simulink model "MPC_lateralStability_IntegratedControl_DesignProgram"  (R2019b)
settings: Solver=VariableStepAuto  StartTime=0.0  StopTime=10.0  RelTol=1e-3
values from neighbouring files (symbols this model uses):
  A = [-4.40211640212  -0.830687830688; 20.8695652174  -5.1867826087]    [general_mpc_test_data.mat]
  B = [1.60846560847  0; 15.8608695652  0.000347826086957]    [general_mpc_test_data.mat]
libraries: mpclib x2
settings Model: Creator=Shouvik Chakraborty  LastModifiedBy=shouv
settings SFSimCC: CustomCodeUndefinedFunction=UseInterfaceOnly

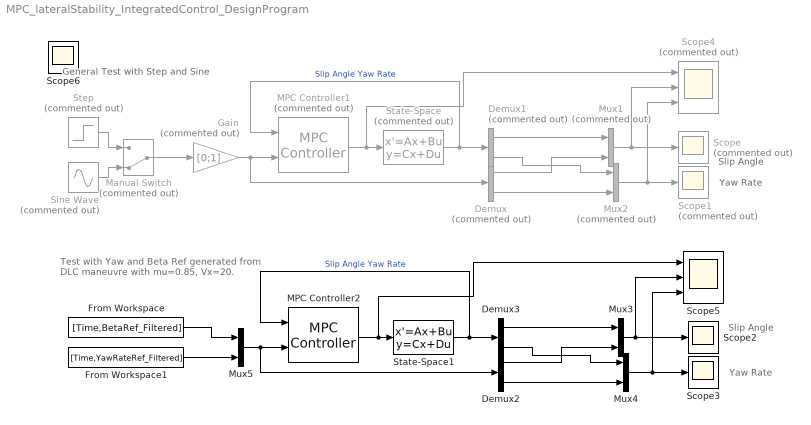
== system MPC_lateralStability_IntegratedControl_DesignProgram ==
  note: Test with Yaw and Beta Ref generated
      | from DLC maneuvre with mu=0.85, Vx=20.
  note: General Test with Step and Sine
  note: Yaw Rate
  note: Slip Angle
  note: Yaw Rate
  note: Slip Angle
  Demux : Demux  Commented=on  Outputs=2
  Demux1 : Demux  Commented=on  Outputs=2
  Demux2 : Demux  Outputs=2
  Demux3 : Demux  Outputs=2
  From Workspace : FromWorkspace  VariableName=[Time,BetaRef_Filtered]  SampleTime=0
  From Workspace1 : FromWorkspace  VariableName=[Time,YawRateRef_Filtered]  SampleTime=0
  Gain : Gain  Commented=on  Gain=[0;1]
  MPC Controller1 : mpclib/MPC Controller  Commented=on  SCDEnableBlockLinearizationSpecification=on  mpcobj=mpcIntegratedControl  is_multiple=0  enable_value=0  return_u0=off  updateMPCinCallerWorkspace=on  md_inport=off  mv_inport=off  uref_inport=off  return_cost=off  return_mvseq=off  return_qpstatus=off  return_xseq=off  return_state=off  return_ovseq=off  state_inport=off  umin_inport=off  umax_inport=off  ymin_inport=off  ymax_inport=off  cc_inport=off  ywt_inport=off  uwt_inport=off  duwt_inport=off  rhoeps_inport=off  pm_inport=off  MaximumP=10  HorizonChoice=FixedHorizon  n_ts=0.025  n_p=3  n_mv=2  n_md=0  n_ud=0  n_mo=2  n_uo=0  BlockDataType=double  SampleTimeInherited=off  switch_inport=off
  MPC Controller2 : mpclib/MPC Controller  SCDEnableBlockLinearizationSpecification=on  mpcobj=mpcIntegratedControl  is_multiple=0  enable_value=0  return_u0=off  updateMPCinCallerWorkspace=on  md_inport=off  mv_inport=off  uref_inport=off  return_cost=off  return_mvseq=off  return_qpstatus=off  return_xseq=off  return_state=off  return_ovseq=off  state_inport=off  umin_inport=off  umax_inport=off  ymin_inport=off  ymax_inport=off  cc_inport=off  ywt_inport=off  uwt_inport=off  duwt_inport=off  rhoeps_inport=off  pm_inport=off  MaximumP=10  HorizonChoice=FixedHorizon  n_ts=0.025  n_p=3  n_mv=2  n_md=0  n_ud=0  n_mo=2  n_uo=0  BlockDataType=double  SampleTimeInherited=off  switch_inport=off
  Manual Switch : ManualSwitch  Commented=on  CurrentSetting=0
  Mux1 : Mux  Commented=on  Inputs=2
  Mux2 : Mux  Commented=on  Inputs=2
  Mux3 : Mux  Inputs=2
  Mux4 : Mux  Inputs=2
  Mux5 : Mux  Inputs=2
  Scope : Scope  Commented=on
  Scope1 : Scope  Commented=on
  Scope2 : Scope
  Scope3 : Scope
  Scope4 : Scope  Commented=on  NumInputPorts=3
  Scope5 : Scope  NumInputPorts=3
  Sine Wave : Sin  Commented=on  SampleTime=0
  State-Space : StateSpace  Commented=on  A=A  B=B  C=eye(2)  D=[0 0;0 0]  InitialCondition=0
  State-Space1 : StateSpace  A=A  B=B  C=eye(2)  D=[0 0;0 0]  InitialCondition=0
  Step : Step  Commented=on  SampleTime=0
  Scope6 : Scope
  wires:
  State-Space/1 -> MPC Controller1/1, Demux1/1  "Slip Angle Yaw Rate"
  Manual Switch/1 -> Gain/1
  Gain/1 -> Demux/1, MPC Controller1/2
  Sine Wave/1 -> Manual Switch/2
  Step/1 -> Manual Switch/1
  MPC Controller1/1 -> Scope4/1, State-Space/1
  Demux1/1 -> Mux1/1
  Demux/1 -> Mux1/2
  Demux1/2 -> Mux2/1
  Demux/2 -> Mux2/2
  Mux1/1 -> Scope4/2, Scope/1
  Mux2/1 -> Scope4/3, Scope1/1
  Mux4/1 -> Scope5/3, Scope3/1
  MPC Controller2/1 -> Scope5/1, State-Space1/1
  Mux5/1 -> Demux2/1, MPC Controller2/2
  Demux2/1 -> Mux3/2
  Demux3/2 -> Mux4/1
  State-Space1/1 -> MPC Controller2/1, Demux3/1  "Slip Angle Yaw Rate"
  Demux3/1 -> Mux3/1
  Mux3/1 -> Scope5/2, Scope2/1
  Demux2/2 -> Mux4/2
  From Workspace/1 -> Mux5/1
  From Workspace1/1 -> Mux5/2
